simulink model "ex04"  (R2015b)
settings: Solver=VariableStepAuto  StartTime=0.0  StopTime=4*T  RelTol=1e-3
values from neighbouring files (symbols this model uses):
  A = 1    [init.m]
  T = 1    [init.m]
settings Model: Creator=Tom  LastModifiedBy=Tom

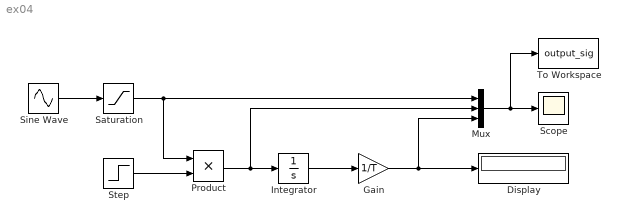
== system ex04 ==
  Display : Display
  Gain : Gain  Gain=1/T
  Integrator : Integrator
  Mux : Mux  Inputs=3
  Product : Product
  Saturation : Saturate  UpperLimit=Inf  LowerLimit=0
  Scope : Scope
  Sine Wave : Sin  Amplitude=A  Frequency=2*pi/T  SampleTime=0
  Step : Step  Time=T  Before=1  After=0  SampleTime=0
  To Workspace : ToWorkspace  VariableName=output_sig  SaveFormat=Structure With Time  SampleTime=-1
  wires:
  Mux/1 -> To Workspace/1, Scope/1
  Sine Wave/1 -> Saturation/1
  Saturation/1 -> Mux/1, Product/1
  Integrator/1 -> Gain/1
  Step/1 -> Product/2
  Product/1 -> Mux/2, Integrator/1
  Gain/1 -> Display/1, Mux/3
